simulink model "milstd_TestEncoderFigure4"  (Simulink 6.0)
settings: Solver=ode45  StartTime=0.0  StopTime=10.0  RelTol=1e-3
libraries: dspobslib x6, dspbuff3 x2, commcnvcod2 x2, commsink2 x2, commrandsrc2 x1, dspsigattribs x1, commsequence2 x1
settings Model: Creator=arodrigu  LastModifiedBy=arodrigu
settings DataIOCC: SignalLoggingName=sigsOut
settings OptimizationCC: BooleanDataType=off
settings DebuggingCC: CheckExecutionContextPreStartOutputMsg=on  CheckExecutionContextRuntimeOutputMsg=on  SolverPrmCheckMsg=none
settings HardwareCC: TargetUnknown=on
settings ModelReferenceCC: UpdateModelReferenceTargets=IfOutOfDate
settings GRTTargetCC: LifeSpan=inf
settings SFSimCC: SFSimApplyToAllLibs=on  SFSimBuildMode=Incremental

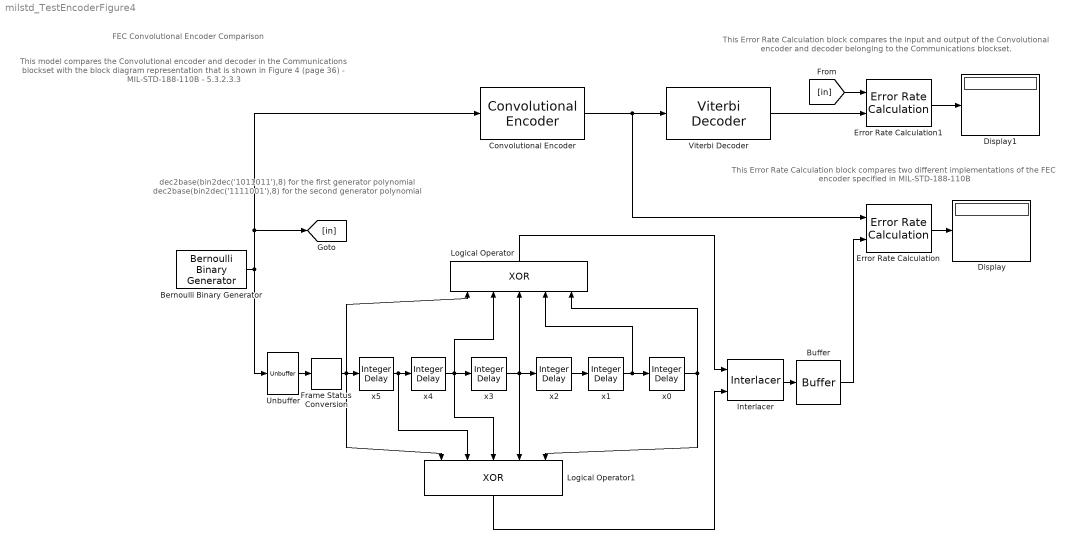
== system milstd_TestEncoderFigure4 ==
  note: FEC Convolutional Encoder Comparison
  note: This model compares the Convolutional encoder and decoder
      | in the Communications blockset with the block diagram representation
      | that is shown in Figure 4 (page 36) - MIL-STD-188-110B - 5.3.2.3.3
  note: dec2base(bin2dec('1011011'),8)  for the first generator polynomial
      | dec2base(bin2dec('1111001'),8)  for the second generator polynomial
  note: This Error Rate Calculation block compares the input and output
      | of the Convolutional encoder and decoder belonging to the
      | Communications blockset.
  note: This Error Rate Calculation block compares two different
      | implementations of the FEC encoder specified in MIL-STD-188-110B
  Bernoulli Binary Generator : commrandsrc2/Bernoulli Binary Generator  P=0  seed=61  Ts=1/100  frameBased=on  sampPerFrame=100  orient=off
  Buffer : dspbuff3/Buffer  N=100*2  V=0  ic=0
  Convolutional Encoder : commcnvcod2/Convolutional Encoder  trellis=poly2trellis(7, [133 171])  reset=None
  Display : Display
  Display1 : Display
  Error Rate Calculation : commsink2/Error Rate Calculation  N=200  st_delay=0  cp_mode=Entire frame  subframe=[]  PMode=Port  WsName=ErrorVec  RsMode2=off  stop=off  numErr=100  maxBits=1e6
  Error Rate Calculation1 : commsink2/Error Rate Calculation  N=34  st_delay=0  cp_mode=Entire frame  subframe=[]  PMode=Port  WsName=ErrorVec  RsMode2=off  stop=off  numErr=100  maxBits=1e6
  Frame Status Conversion : dspsigattribs/Frame Status Conversion  growRefPort=off  outframe=Frame-based
  Interlacer : commsequence2/Interlacer
  Logical Operator : Logic  Orientation=up  Operator=XOR  Inputs=5  AllPortsSameDT=off
  Logical Operator1 : Logic  Orientation=down  Operator=XOR  Inputs=5  AllPortsSameDT=off
  Unbuffer : dspbuff3/Unbuffer  ic=0
  Viterbi Decoder : commcnvcod2/Viterbi Decoder  trellis=poly2trellis(7, [133 171])  dectype=Hard Decision  nsdecb=4  tbdepth=34  opmode=Continuous  reset=off
  x{0..5} (6 alike) : dspobslib/Integer Delay  delay=1  ic=0  reset_popup=None
  wires:
  x5/1 -> x4/1, Logical Operator1/2
  x4/1 -> Logical Operator/2, x3/1, Logical Operator1/3
  x3/1 -> x2/1, Logical Operator/3, Logical Operator1/4
  x2/1 -> x1/1
  x1/1 -> x0/1, Logical Operator/4
  x0/1 -> Logical Operator/5, Logical Operator1/5
  Logical Operator/1 -> Interlacer/1
  Logical Operator1/1 -> Interlacer/2
  Bernoulli Binary Generator/1 -> Unbuffer/1, Convolutional Encoder/1, [in]
  Unbuffer/1 -> Frame Status Conversion/1
  Frame Status Conversion/1 -> x5/1, Logical Operator/1, Logical Operator1/1
  Error Rate Calculation/1 -> Display/1
  Convolutional Encoder/1 -> Error Rate Calculation/1, Viterbi Decoder/1
  Interlacer/1 -> Buffer/1
  Buffer/1 -> Error Rate Calculation/2
  Error Rate Calculation1/1 -> Display1/1
  Viterbi Decoder/1 -> Error Rate Calculation1/2
  [in] -> Error Rate Calculation1/1
